simulink model "lyskawaProject_si_tr"  (R2023b)
settings: Solver=VariableStepAuto  StartTime=startTime  StopTime=stopTime  MaxStep=maxStepSize  RelTol=1e-3
values from neighbouring files (symbols this model uses):
  dTk = 0    [lyskawaProject.m]    (also in nieliniowe.m; rStanu.m; transmitancje.m)
  dTz = 5    [lyskawaProject.m]    (also in nieliniowe.m = 0; rStanu.m = 2; transmitancje.m = 2)
  LTk1 = [Cvp*a, a*(a+Kp+K2)]    [lyskawaProject.m]    (also in transmitancje.m)
  LTk2 = a*(a+Kp)    (= 831168.831169)    [lyskawaProject.m]    (also in transmitancje.m = a*(a+Kp))
  LTz1 = [K1*Cvp, K1*a+K1*Kp+K1*K2+Kp*K2]    [lyskawaProject.m]    (also in transmitancje.m)
  LTz2 = [K2*Cvw, K2*a+K2*K1+K2*Kp+K1*a+K1*Kp]    [lyskawaProject.m]    (also in transmitancje.m)
  M = [Cvw*Cvp, Cvw*(a+Kp+K2)+Cvp*(a+K1+Kp), a*(a+K1+K2+Kp)+K1*Kp+K1*K2+Kp*K2]    [lyskawaProject.m]    (also in transmitancje.m)
  t0 = 10    [lyskawaProject.m]    (also in nieliniowe.m = 100; rStanu.m = 100; test2.m; transmitancje.m = 100)
  Tp0 = x(2)    [lyskawaProject.m]    (also in nieliniowe.m; rStanu.m; test2.m = 10; transmitancje.m)
  Tw0 = x(1)    [lyskawaProject.m]    (also in nieliniowe.m; rStanu.m; transmitancje.m)
settings Model: Creator=aleklyskawa  LastModifiedBy=aleklyskawa

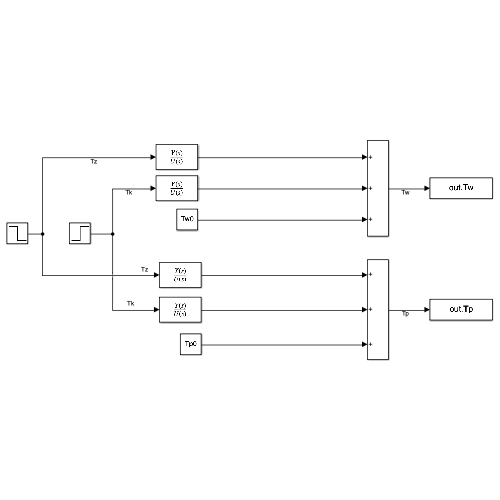
[thumbnail: Simulink's stored preview of the top-level diagram]
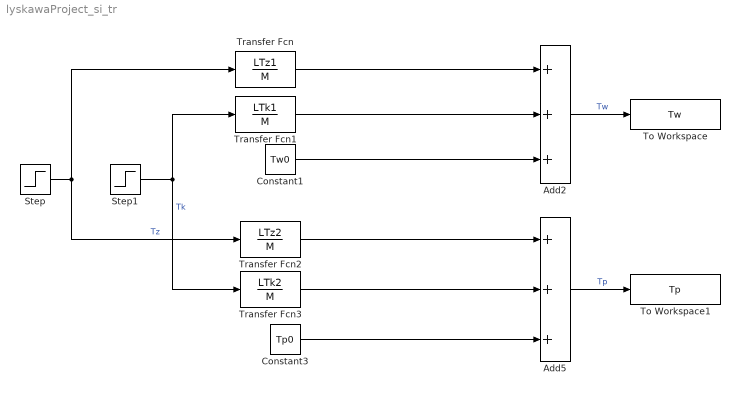
== system lyskawaProject_si_tr ==
  Add2 : Sum  Inputs=+++
  Add5 : Sum  Inputs=+++
  Constant1 : Constant  Value=Tw0
  Constant3 : Constant  Value=Tp0
  Step : Step  Time=t0  After=dTz  SampleTime=0
  Step1 : Step  Time=t0  After=dTk  SampleTime=0
  To Workspace : ToWorkspace  VariableName=Tw  SampleTime=-1
  To Workspace1 : ToWorkspace  VariableName=Tp  SampleTime=-1
  Transfer Fcn : TransferFcn  Numerator=LTz1  Denominator=M
  Transfer Fcn1 : TransferFcn  Numerator=LTk1  Denominator=M
  Transfer Fcn2 : TransferFcn  Numerator=LTz2  Denominator=M
  Transfer Fcn3 : TransferFcn  Numerator=LTk2  Denominator=M
  wires:
  Add5/1 -> To Workspace1/1  "Tp"
  Constant3/1 -> Add5/3
  Transfer Fcn/1 -> Add2/1
  Step1/1 -> Transfer Fcn3/1, Transfer Fcn1/1  "Tk"
  Transfer Fcn3/1 -> Add5/2
  Transfer Fcn1/1 -> Add2/2
  Transfer Fcn2/1 -> Add5/1
  Add2/1 -> To Workspace/1  "Tw"
  Constant1/1 -> Add2/3
  Step/1 -> Transfer Fcn2/1, Transfer Fcn/1  "Tz"
